simulink model "Cathode_Simscape_Model"  (R2023a)
settings: Solver=VariableStepAuto  StartTime=0.0  StopTime=500  RelTol=1e-3
undefined symbols (not defined in the file or in its folder): sigbuilder_block
libraries: fl_lib x55, nesl_utility x45, SimscapeFluids_lib x15
(part 1 of 3)
settings Model: Creator=mahesh.kumar  LastModifiedBy=mahesh.kumar

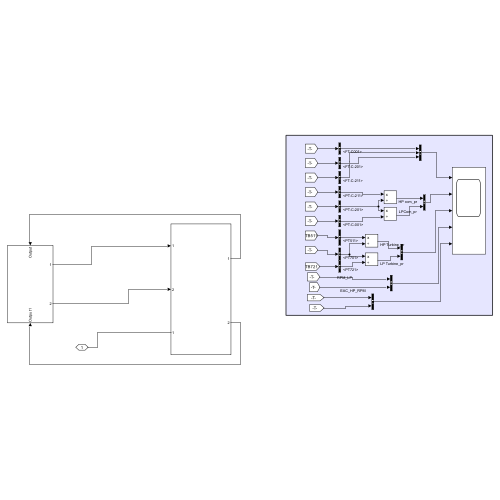
[thumbnail: Simulink's stored preview of the top-level diagram]
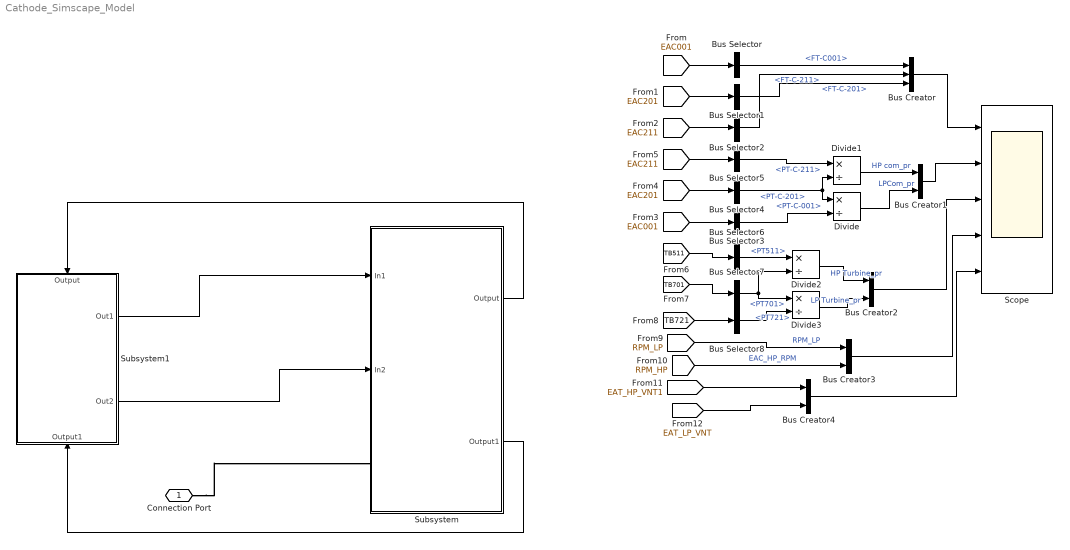
== system Cathode_Simscape_Model ==
  Bus Creator : BusCreator  Inputs=3
  Bus Creator{1..4} (4 alike) : BusCreator  Inputs=2
  Bus Selector : BusSelector  OutputSignals=FT-C001
  Bus Selector1 : BusSelector  OutputSignals=FT-C-201
  Bus Selector2 : BusSelector  OutputSignals=FT-C-211
  Bus Selector3 : BusSelector  OutputSignals=PT-C-001
  Bus Selector4 : BusSelector  OutputSignals=PT-C-201
  Bus Selector5 : BusSelector  OutputSignals=PT-C-211
  Bus Selector6 : BusSelector  OutputSignals=PT511
  Bus Selector7 : BusSelector  OutputSignals=PT701
  Bus Selector8 : BusSelector  OutputSignals=PT721
  Divide{,1..3} (4 alike) : Product  Inputs=*/
  Scope : Scope  NumInputPorts=5
  Subsystem : Subsystem
  Subsystem1 : Subsystem
      settings: PortSchema="{\"entries\":[{\"content\":{\"sides\":[{\"content\":{},\"type\":\"ConnectorPlacement.EquallySpacedRectSide\",\"uuid\":\"984249b6-2700-4899-8357-f545c62d10ef\"},{\"content\":{\"connectorIds\":[\"Out1\",\"Out2\"],\"side\":\"RIGHT\"},\"type\":\"ConnectorPlacement.EquallySpacedRectSide\",\"uuid\":\"0a8907d5-2e85-49aa-bb23-8dd611067149\"},{\"content\":{\"connectorIds\":[\"In1\"],\"side\":\"TOP\"},\"type\":\"ConnectorPlacement.EquallySpacedRectSide\",\"uuid\":\"e00e54d0-6dbf-429f-9506-ec6eaddd1938\"},{\"content\":{\"connectorIds\":[\"In2\"],\"side\":\"BOTTOM\"},\"type\":\"ConnectorPlacement.EquallySpacedRectSide\",\"uuid\":\"b22db3dd-63f8-4b6d-a56a-cf8370c91cba\"}]},\"type\":\"ConnectorPlacement.EquallySpacedConnector\",\"uuid\":\"9582d771-9072-4842-b99f-8327be8cf876\"}],\"packageUris\":[\"http://schema.mathworks.com/mf0/Connector/R2020b\"],\"version\":\"1.0\"}"
  Connection Port : PMIOPort  Side=Left
  wires:
  Subsystem1/1(Out1) -> Subsystem/1(In1)
  Subsystem1/2(Out2) -> Subsystem/2(In2)
  Subsystem/1(Output) -> Subsystem1/1(Output)
  [EAC001] -> Bus Selector/1
  [EAC201] -> Bus Selector1/1
  [EAC211] -> Bus Selector2/1
  Bus Selector/1 -> Bus Creator/1  "<FT-C001>"
  Bus Selector1/1 -> Bus Creator/3  "<FT-C-201>"
  Bus Selector2/1 -> Bus Creator/2  "<FT-C-211>"
  Bus Selector4/1 -> Divide/1, Divide1/2  "<PT-C-201>"
  [EAC001] -> Bus Selector3/1
  [EAC201] -> Bus Selector4/1
  Bus Selector3/1 -> Divide/2  "<PT-C-001>"
  [EAC211] -> Bus Selector5/1
  Bus Selector5/1 -> Divide1/1  "<PT-C-211>"
  Divide1/1 -> Bus Creator1/1  "HP com_pr"
  Divide/1 -> Bus Creator1/2  "LPCom_pr"
  [TB511] -> Bus Selector6/1
  [TB701] -> Bus Selector7/1
  Bus Selector6/1 -> Divide2/1  "<PT511>"
  Bus Selector7/1 -> Divide3/1, Divide2/2  "<PT701>"
  [TB721] -> Bus Selector8/1
  Bus Selector8/1 -> Divide3/2  "<PT721>"
  Divide2/1 -> Bus Creator2/1  "HP Turbine_pr"
  Divide3/1 -> Bus Creator2/2  "LP Turbine_pr"
  Subsystem/2(Output1) -> Subsystem1/2(Output1)
  Bus Creator/1 -> Scope/1
  Bus Creator1/1 -> Scope/2
  Bus Creator2/1 -> Scope/3
  [RPM_LP] -> Bus Creator3/1  "RPM_LP"
  [RPM_HP] -> Bus Creator3/2  "EAC_HP_RPM"
  Bus Creator3/1 -> Scope/4
  [EAT_HP_VNT1] -> Bus Creator4/1
  [EAT_LP_VNT] -> Bus Creator4/2
  Bus Creator4/1 -> Scope/5
  connections:
  Connection Port/RConn1 -- Subsystem/LConn1

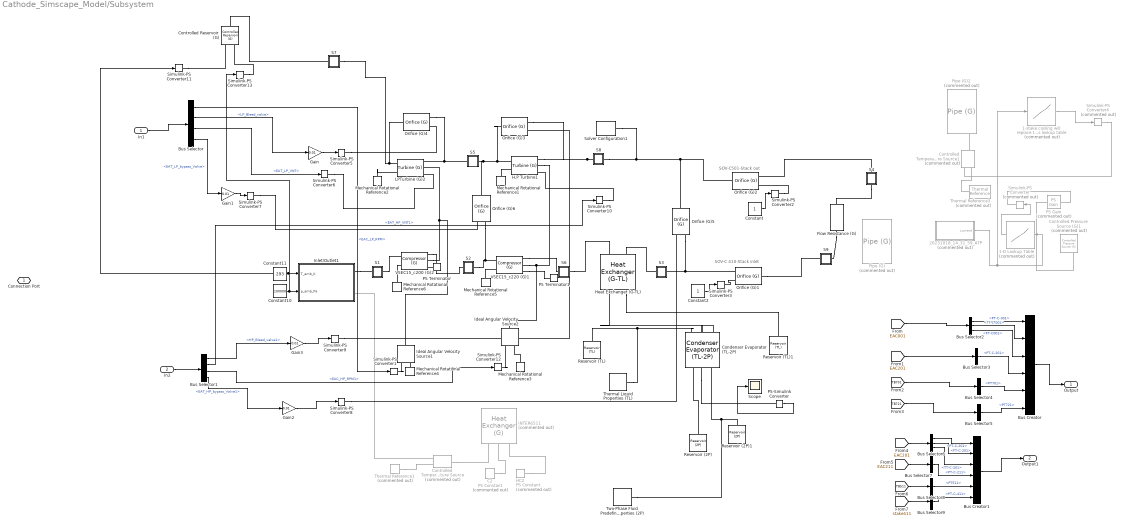
== system Cathode_Simscape_Model/Subsystem ==
  note: SOV-C 410-Stack inlet
  note: SOV-C501-Stack out
  In1 : Inport
  In2 : Inport  Port=2
  1-D Lookup Table : Lookup_n-D  Commented=on  NumberOfTableDimensions=1  BreakpointsForDimension1=[50;100;150;200;250;300;350;400;450;500;550;600]  Table=[49.4;55;69.9;83;109;105;153;173;174;220;230;0]  InternalRulePriority=Speed  RndMeth=Simplest
  1-stake cooling will replace this lookup table : Lookup_n-D  Commented=on  NumberOfTableDimensions=1  BreakpointsForDimension1=[0;50;100;200;400]  Table=[312;322;332;342;352]  InternalRulePriority=Speed  RndMeth=Simplest
  20231018_14_31_59_ATP : Subsystem  Tag=STV Subsys  Commented=on  LoadFcn=sigbuilder_block('load');  StartFcn=sigbuilder_block('start');  StopFcn=sigbuilder_block('stop');  ClipboardFcn=sigbuilder_block('clipboard');  mask(Sigbuilder block){tuvar=[0:10]}
      mask help: Simulink:masks:SigbuilderBlock_MD
      mask init:
      | if ~strcmp(get_param(bdroot(gcbh),'SimulationStatus'),'stopped') tuvar = sigbuilder_block('maskInit'); end
      settings: CopyFcn=sigbuilder_block('copy');  DeleteFcn=sigbuilder_block('delete');  ModelCloseFcn=sigbuilder_block('modelClose');  PreSaveFcn=sigbuilder_block('preSave');  PauseFcn=sigbuilder_block('pause');  ContinueFcn=sigbuilder_block('continue');  NameChangeFcn=sigbuilder_block('namechange');  OpenFcn=sigbuilder_block('open',[368.25 148.5 938.25 516 ]);  CloseFcn=sigbuilder_block('close');
      mask Display: plot(0, 0, 100, 100,[2, 2, 32, 32, 2], [68, 8, 8, 68, 68],[32, 2], [38, 38], [32, 19, 2],[53, 60, 44], [32, 17, 17, 2],[16, 16, 31, 31]);txt = getActiveGroup(gcbh);text(2, 100, txt,'verticalAlignment', 'top');
  Bus Creator : BusCreator  Inputs=6
  Bus Creator1 : BusCreator  Inputs=6
  Bus Selector : BusSelector  OutputSignals=EAC_LP_RPM,LP_Bleed_valve,EAT_LP_VNT,EAT_LP_bypass_Valve
  Bus Selector1 : BusSelector  OutputSignals=HP_Bleed_valve1,EAT_HP_VNT1,EAC_HP_RPM1,EAT_HP_bypass_Valve1
  Bus Selector2 : BusSelector  OutputSignals=PT-C-001,TT-C-001,FT-C001
  Bus Selector3 : BusSelector  OutputSignals=PT-C-201
  Bus Selector4 : BusSelector  OutputSignals=PT701
  Bus Selector5 : BusSelector  OutputSignals=PT721
  Bus Selector6 : BusSelector  OutputSignals=PT-C-201,FT-C-201,TT-C-201
  Bus Selector7 : BusSelector  OutputSignals=PT-C-211
  Bus Selector8 : BusSelector  OutputSignals=PT511
  Bus Selector9 : BusSelector  OutputSignals=PT-C-411
  C2 : fl_lib/Physical Signals/Sources/PS Constant  Commented=on  constant=12361
  Condenser Evaporator (TL-2P) : SimscapeFluids_lib/Fluid Network Interfaces/Heat Exchangers/Condenser Evaporator (TL-2P)  flow_arrangement=fluids.interfaces.heat_exchangers.enum.FlowArrangementTL2P.Cross  cross_flow_arrangement=fluids.interfaces.heat_exchangers.enum.CrossFlowArrangementTL2P.UnmixedUnmixed  R_wall=0 K/kW  area_A1=0.01 m^2  area_B1=0.01 m^2  area_A2=0.01 m^2  area_B2=0.01 m^2  flow_geometry_TL=fluids.interfaces.heat_exchangers.enum.FlowGeometryTL.InsideTubes  tube_num_TL=25  tube_length_TL=1 m  tube_cross_section_TL=fluids.interfaces.heat_exchangers.enum.TubeCrossSection.Circular  tube_diameter_TL=0.05 m  tube_width_TL=0.05 m  tube_height_TL=0.05 m  tube_inner_diameter_TL=0.05 m  tube_outer_diameter_TL=0.1 m  tube_flow_area_TL=0.002 m^2  tube_wetted_perimeter_TL=0.15 m  tube_heat_perimeter_TL=0.15 m  tube_pressure_loss_spec_TL=fluids.interfaces.heat_exchangers.enum.TubePressureLossSpec.Haaland  tube_loss_coeff_TL=10  tube_local_pressure_loss_spec_TL=fluids.thermal_liquid.pipes_fittings.enum.LocalLossSpec.AggregateLength  tube_length_add_TL=0.1 m  tube_local_loss_coefficient_TL=0.1  tube_roughness_pressure_TL=15e-6 m  tube_Re_lam_pressure_TL=2000  tube_Re_tur_pressure_TL=4000  tube_shape_factor_generic_TL=64  tube_heat_coeff_spec_TL=fluids.interfaces.heat_exchangers.enum.TubeHeatCoeffSpec.Gneilinski  tube_colburn_coeff_TL=[.023, .8, .33]  tube_roughness_heat_TL=15e-6 m  tube_Re_lam_heat_TL=2000  tube_Re_tur_heat_TL=4000  tube_Nu_lam_generic_TL=3.66  bank_arrangement_TL=fluids.interfaces.heat_exchangers.enum.BankArrangement.Inline  bank_num_rows_TL=5  bank_tubes_per_row_TL=5  bank_width_TL=1 m  bank_tube_diameter_TL=0.05 m  bank_longitudinal_pitch_TL=0.15 m  bank_transverse_pitch_TL=0.15 m  bank_pressure_loss_spec_TL=fluids.interfaces.heat_exchangers.enum.BankPressureLossSpec.Martin  bank_euler_TL=10  bank_heat_coeff_spec_TL=fluids.interfaces.heat_exchangers.enum.BankHeatCoeffSpec.Martin  bank_colburn_coeff_TL=[.27, .63, .36]  generic_flow_area_TL=0.01 m^2  generic_heat_area_TL=2 m^2  generic_volume_TL=0.05 m^3  generic_loss_coeff_TL=10  generic_colburn_coeff_TL=[.023, .8, .33]  fouling_factor_TL=0.1 K*m^2/kW  fin_area_TL=0 m^2  fin_efficiency_TL=0.5  p_init_TL=0.101325 MPa  T_init_TL=293.15 K  tube_num_2P=25  tube_length_2P=1 m  tube_cross_section_2P=fluids.interfaces.heat_exchangers.enum.TubeCrossSection.Circular  tube_diameter_2P=0.05 m  tube_width_2P=0.05 m  tube_height_2P=0.05 m  tube_inner_diameter_2P=0.05 m  tube_outer_diameter_2P=0.1 m  tube_flow_area_2P=0.002 m^2  tube_wetted_perimeter_2P=0.15 m  tube_heat_perimeter_2P=0.15 m  tube_pressure_loss_spec_2P=fluids.interfaces.heat_exchangers.enum.TubePressureLossSpec2P.Haaland  tube_loss_coeff_2P=10  tube_local_pressure_loss_spec_2P=fluids.two_phase_fluid.pipes_fittings.enum.LocalLossSpec.AggregateLength  tube_length_add_2P=0.1 m  tube_local_loss_coefficient_2P=0.1  tube_roughness_pressure_2P=15e-6 m  tube_Re_lam_pressure_2P=2000  tube_Re_tur_pressure_2P=4000  tube_shape_factor_generic_2P=64  tube_heat_coeff_spec_2P=fluids.interfaces.heat_exchangers.enum.TubeHeatCoeffSpec2P.GneilinskiCavalliniZecchin  tube_colburn_coeff_liq_2P=[.023, .8, .33]  tube_colburn_coeff_mix_2P=[.05, .8, .33]  tube_colburn_coeff_vap_2P=[.023, .8, .33]  tube_roughness_heat_2P=15e-6 m  tube_Re_lam_heat_2P=2000  tube_Re_tur_heat_2P=4000  tube_Nu_lam_generic_2P=3.66  fouling_factor_2P=0.1 K*m^2/kW  fin_area_2P=0 m^2  fin_efficiency_2P=0.5  energy_spec_2P=foundation.enum.energy_spec.temperature  p_init_2P=0.101325 MPa  T_init_2P=293.15 K  x_init_2P=0.5  alpha_init_2P=0.5  h_init_2P=1500 kJ/kg  u_init_2P=1500 kJ/kg
      settings: InternalSimscapePortConfiguration="{\"Bottom\":[],\"Left\":[{\"id\":\"A1\",\"label\":\"A1\",\"type\":\"foundation.thermal_liquid.thermal_liquid\"},{\"id\":\"B1\",\"label\":\"B1\",\"type\":\"foundation.thermal_liquid.thermal_liquid\"}],\"Right\":[{\"id\":\"A2\",\"label\":\"A2\",\"type\":\"foundation.two_phase_fluid.two_phase_fluid\"},{\"id\":\"B2\",\"label\":\"B2\",\"type\":\"foundation.two_phase_fluid.two_phase_fluid\"}],\"Top\":[{\"id\":\"Z\",\"label\":\"Z\",\"type\":\"output\"}]}"
  Constant : Constant
  Constant10 : Constant  Value=100000
  Constant11 : Constant  Value=293
  Constant2 : Constant
  Controlled Temperature Source : fl_lib/Thermal/Thermal Sources/Controlled Temperature Source  Commented=on
  Controlled Temperature Source1 : fl_lib/Thermal/Thermal Sources/Controlled Temperature Source  Commented=on
  Controlled Pressure Source (G)1 : fl_lib/Gas/Sources/Controlled Pressure Source (G)  Commented=on  power_spec=foundation.enum.power_spec.none  area_A=0.01 m^2  area_B=0.01 m^2
      settings: InternalSimscapePortConfiguration="{\"Bottom\":[],\"Left\":[{\"id\":\"A\",\"label\":\"A\",\"type\":\"foundation.gas.gas\"},{\"id\":\"P\",\"label\":\"P\",\"type\":\"input\"}],\"Right\":[{\"id\":\"B\",\"label\":\"B\",\"type\":\"foundation.gas.gas\"}],\"Top\":[]}"
  Controlled Reservoir (G) : fl_lib/Gas/Elements/Controlled Reservoir (G)  area_A=0.002 m^2
      settings: InternalSimscapePortConfiguration="{\"Bottom\":[],\"Left\":[{\"id\":\"A\",\"label\":\"A\",\"type\":\"foundation.gas.gas\"}],\"Right\":[{\"id\":\"T_in\",\"label\":\"T\",\"type\":\"input\"},{\"id\":\"p_in\",\"label\":\"P\",\"type\":\"input\"}],\"Top\":[]}"
  Flow Resistance (G) : fl_lib/Gas/Elements/Flow Resistance (G)  delta_p_nominal=20000 Pa  mdot_nominal=0.1 kg/s  rho_nominal=0 kg/m^3  area=0.002 m^2  laminar_fraction=1e-3
      settings: InternalSimscapePortConfiguration="{\"Bottom\":[],\"Left\":[{\"id\":\"A\",\"label\":\"A\",\"type\":\"foundation.gas.gas\"}],\"Right\":[{\"id\":\"B\",\"label\":\"B\",\"type\":\"foundation.gas.gas\"}],\"Top\":[]}"
  Gain{,1..3} (4 alike) : Gain  Gain=0.01
  H.P Turbine1 : SimscapeFluids_lib/Gas/Turbomachinery/Turbine (G)  parameterization=fluids.gas.turbomachinery.enum.TurbineParameterization.Tabulated1D  omega_TLU_2="[40000, 60000, 80000,  100000, 120000] rpm"  variable_nozzle=true  min_nozzle_opening=1e-3  max_nozzle_opening=1  pr_nom=2  mdot_nom=48 kg/s  pr_mdot_TLU=[1.02750530846485, 1.10195466284075, 1.21807977044476, 1.39993572453372, 1.59797761836442, 1.85853658536585]  mdot_TLU=[37.7618364418938, 59.6556671449067, 79.3400286944046, 95.2080344332855, 105.652797704448, 112.682926829268] g/s  pr_mdot_TLU_2=|  mdot_TLU_2=|  efficiency_constant=0.8  pr_eta_TLU=[1.02750530846485, 1.10195466284075, 1.21807977044476, 1.39993572453372, 1.59797761836442, 1.85853658536585]  eta_TLU=[0.500,0.473,0.375,0.337,0.310,0.290]  pr_eta_TLU_2=|  eta_TLU_2=|  p_reference=1 bar  T_reference=293 K  mechanical_efficiency=0.98  area_A=0.002 m^2  area_B=0.002 m^2
      pr_mdot_TLU_2=|
      | [1.02750530846485 1.10195466284075 1.21807977044476 1.39993572453372 1.59797761836442 1.85853658536585;
      | 1.04528436154950 1.18521664275466 1.44373486370158 1.67865939741750 1.86888723098996 2.13912883787661; 
      | 1.05182209469154 1.19671965566714 1.42019626972740 1.67269325681492 1.95725911047346 2.27246599713056; 
      | 1.05523558106169 1.20345710186514 1.43823012912482 1.69874777618364 1.91463070301291 2.21694806312769; 
      | 1.06813888091822 1.31716040172166 1.53931248206600 1.75356786226686 2.00627144906743 2.20147144906743]
      mdot_TLU_2=|
      | [37.7618364418938 59.6556671449067 79.3400286944046 95.2080344332855 105.652797704448 112.682926829268;
      | 32.5394548063128 57.8479196556671 77.7331420373027 85.7675753228121 90.7890961262554 95.4088952654233; 
      | 28.5222381635581 49.0100430416069 64.2754662840746 73.1133428981349 79.9426111908178 79.7417503586801; 
      | 22.2955523672884 39.1678622668580 51.6212338593974 59.8565279770445 63.2711621233860 65.6814921090387; 
      | 19.2826398852224 36.1549497847920 43.3859397417504 47.6040172166428 50.4160688665710 50.4160688665710] g/s
      pr_eta_TLU_2=|
      | [1.02750530846485 1.10195466284075 1.21807977044476 1.39993572453372 1.59797761836442 1.85853658536585;
      | 1.04528436154950 1.18521664275466 1.44373486370158 1.67865939741750 1.86888723098996 2.13912883787661; 
      | 1.05182209469154 1.19671965566714 1.42019626972740 1.67269325681492 1.95725911047346 2.27246599713056; 
      | 1.05523558106169 1.20345710186514 1.43823012912482 1.69874777618364 1.91463070301291 2.21694806312769; 
      | 1.06813888091822 1.31716040172166 1.53931248206600 1.75356786226686 2.00627144906743 2.20147144906743]
      eta_TLU_2=|
      | [0.7 0.7 0.7 0.7 0.7 0.7;
      |   0.7 0.7 0.7 0.7 0.7 0.7;
      |    0.7 0.7 0.7 0.7 0.7 0.7;
      |    0.7 0.7 0.7 0.7 0.7 0.7 ;  0.7 0.7 0.7 0.7 0.7 0.7 ]
      settings: InternalSimscapePortConfiguration="{\"Bottom\":[],\"Left\":[{\"id\":\"A\",\"label\":\"A\",\"type\":\"foundation.gas.gas\"},{\"id\":\"R\",\"label\":\"R\",\"type\":\"foundation.mechanical.rotational.rotational\"},{\"id\":\"VN\",\"label\":\"VN\",\"type\":\"input\"}],\"Right\":[{\"id\":\"B\",\"label\":\"B\",\"type\":\"foundation.gas.gas\"},{\"id\":\"C\",\"label\":\"C\",\"type\":\"foundation.mechanical.rotational.rotational\"}],\"Top\":[]}"
  HC2 : fl_lib/Physical Signals/Sources/PS Constant  Commented=on  constant=3981.072
  Heat Exchanger (G-TL) : SimscapeFluids_lib/Fluid Network Interfaces/Heat Exchangers/Heat Exchanger (G-TL)  hex_type=fluids.interfaces.enum.flow_arrangement_spec.parallel_counter  shell_num=1  cross_type=fluids.interfaces.enum.cross_flow_heat_exchanger_G_TL_spec.mixed_mixed  NTU_TLU=[.5, 1, 2, 3, 4, 5]  CR_TLU=[0, .25, .5, .75, 1]  eff_TLU=[.3, .3, .3, .3, .3; .6, .55, .5, .47, .43; .85, .76, .68, .61, .55; .94, .83, .72, .65, .58; .98, .86, .75, .66, .58; .99, .86, .75, .66, .58]  wall_thermal_dynamics=simscape.enum.onoff.off  thermal_mass_wall=447 J/K  R_wall=1.6e-4 K/W  min_flow_area_1=0.01 m^2  Dh_press_1=0.1 m  gas_volume_1=0.01 m^3  Re_lam_1=2000  Re_tur_1=4000  pressure_loss_spec_1=fluids.interfaces.enum.pressure_loss_spec.constant  pressure_loss_coeff_1=0.1  length_press_1=1 m  length_add_1=0.1 m  roughness_1=15e-6 m  Re_friction_TLU_1=[400, 1000, 1500, 3000, 4000, 6000, 10000, 20000, 40000, 60000, 100000, 100000000]  friction_factor_TLU_1=[.264, .112, .071, .0417, .0387, .0268, .025, .0232, .0226, .022, .0214, .0214]  shape_factor_1=64  Re_Euler_TLU_1=[50, 500, 1000, 2000]  Euler_TLU_1=[4.4505, .6864, .4791, .3755]  heat_transfer_spec_1=fluids.interfaces.enum.heat_transfer_spec.constant  heat_transfer_area_1=0.4 m^2  heat_coeff_1=100 W/(K*m^2)  length_heat_1=1 m  Nu_lam_1=3.66  Re_Colburn_TLU_1=[100, 150, 1000]  Colburn_factor_TLU_1=[.019, .013, .002]  Re_Nu_TLU_1=[100, 150, 1000]  Pr_Nu_TLU_1=[1, 10]  Nu_TLU_1=[3.72, 4.21; 3.75, 4.44; 4.21, 7.15]  fouling_factor_1=1e-4 K*m^2/W  mdot_threshold_1=1e-6 kg/s  min_heat_coeff_1=5 W/(K*m^2)  min_flow_area_2=0.00075 m^2  Dh_press_2=0.1 m  liquid_volume_2=0.01 m^3  Re_lam_2=2000  Re_tur_2=4000  pressure_loss_spec_2=fluids.interfaces.enum.pressure_loss_spec.constant  pressure_loss_coeff_2=0.1  length_press_2=1 m  length_add_2=0.1 m  roughness_2=15e-6 m  Re_friction_TLU_2=[400, 1000, 1500, 3000, 4000, 6000, 10000, 20000, 40000, 60000, 100000, 100000000]  friction_factor_TLU_2=[.264, .112, .071, .0417, .0387, .0268, .025, .0232, .0226, .022, .0214, .0214]  shape_factor_2=64  Re_Euler_TLU_2=[50, 500, 1000, 2000]  Euler_TLU_2=[4.4505, .6864, .4791, .3755]  heat_transfer_spec_2=fluids.interfaces.enum.heat_transfer_spec.constant  heat_transfer_area_2=0.4 m^2  heat_coeff_2=100 W/(K*m^2)  length_heat_2=1 m  Nu_lam_2=3.66  Re_Colburn_TLU_2=[100, 150, 1000]  Colburn_factor_TLU_2=[.019, .013, .002]  Re_Nu_TLU_2=[100, 150, 1000]  Pr_Nu_TLU_2=[1, 10]  Nu_TLU_2=[3.72, 4.21; 3.75, 4.44; 4.21, 7.15]  fouling_factor_2=1e-4 K*m^2/W  min_heat_coeff_2=5 W/(K*m^2)  T0_1=293.15 K  p0_1=0.101325 MPa  dynamic_compressibility_2=simscape.enum.onoff.on  T0_2=293.15 K  p0_2=0.101325 MPa  mdot1_TLU=[.3, .5, .6, .7, 1, 1.4, 1.9, 2.3] kg/s  mdot2_TLU=[.3, .5, 1, 1.3, 1.7, 2, 2.6, 3.3] kg/s  SD_TLU=[.324, .3533, .404, .4253, .4333, .4373, .4453, .4533; .3813, .424, .496, .5307, .544, .5547, .5693, .5787; .4267, .4827, .5813, .6173, .6413, .6573, .672, .6827; .4613, .528, .64, .6987, .7267, .7467, .7707, .7853; .5533, .6467, .8227, .928, .9853, 1.0187, 1.0653, 1.0973; .58, .688, .8853, 1.0147, 1.08, 1.124, 1.176, 1.2147; .624, .7467, .992, 1.148, 1.244, 1.304, 1.3773, 1.4267; .656, .7907, 1.0667, 1.26, 1.376, 1.452, 1.548, 1.612] kW/K  Q_check=fluids.interfaces.enum.SD_max_check.warning  mdot_dp_TLU_1=[.3, .5, 1, 1.5, 2, 2.5] kg/s  p_diff_TLU_1=[3, 5, 10, 25, 35, 50] * 1e-3 MPa  T_ref_in_1=293.15 K  p_ref_in_1=0.101325 MPa  area_1=0.01 m^2  mdot_dp_TLU_2=[.3, .5, 1, 1.5, 2, 2.5] kg/s  p_diff_TLU_2=[3, 5, 10, 25, 35, 50] * 1e-3 MPa  T_ref_in_2=293.15 K  p_ref_in_2=0.101325 MPa  mdot_threshold_2=1e-3 kg/s  area_2=0.01 m^2
      settings: InternalSimscapePortConfiguration="{\"Bottom\":[],\"Left\":[{\"id\":\"A1\",\"label\":\"A1\",\"type\":\"foundation.gas.gas\"},{\"id\":\"B1\",\"label\":\"B1\",\"type\":\"foundation.gas.gas\"}],\"Right\":[{\"id\":\"A2\",\"label\":\"A2\",\"type\":\"foundation.thermal_liquid.thermal_liquid\"},{\"id\":\"B2\",\"label\":\"B2\",\"type\":\"foundation.thermal_liquid.thermal_liquid\"}],\"Top\":[]}"
  INTER6511 : SimscapeFluids_lib/Fluid Network Interfaces/Heat Exchangers/Heat Exchanger (G)  Commented=on  hex_type=fluids.interfaces.enum.flow_arrangement_spec.cross_flow  shell_num=1  cross_type=fluids.interfaces.enum.cross_flow_heat_exchanger_G_spec.unmixed_mixed  NTU_TLU=[.5, 1, 2, 3, 4, 5]  CR_TLU=[0, .25, .5, .75, 1]  eff_TLU=[.3, .3, .3, .3, .3; .6, .55, .5, .47, .43; .85, .76, .68, .61, .55; .94, .83, .72, .65, .58; .98, .86, .75, .66, .58; .99, .86, .75, .66, .58]  R_wall=0.00016331 K/W  min_flow_area_1=.00075 m^2  Dh_press_1=0.0028302 m  gas_volume_1=0.0003375 m^3  Re_lam_1=2000  Re_tur_1=4000  pressure_loss_spec_1=fluids.interfaces.enum.pressure_loss_spec.constant  pressure_loss_coeff_1=0.05  length_press_1=1 m  length_add_1=0.1 m  roughness_1=15e-6 m  Re_friction_TLU_1=[400, 1000, 1500, 3000, 4000, 6000, 10000, 20000, 40000, 60000, 100000, 100000000]  friction_factor_TLU_1=[.264, .112, .071, .0417, .0387, .0268, .025, .0232, .0226, .022, .0214, .0214]  shape_factor_1=64  Re_Euler_TLU_1=[50, 500, 1000, 2000]  Euler_TLU_1=[4.4505, .6864, .4791, .3755]  heat_transfer_spec_1=fluids.interfaces.enum.heat_transfer_spec.constant  heat_transfer_area_1=0.45 m^2  heat_coeff_1=405 W/(K*m^2)  length_heat_1=1 m  Nu_lam_1=3.66  Re_Colburn_TLU_1=[100, 150, 1000]  Colburn_factor_TLU_1=[.019, .013, .002]  Re_Nu_TLU_1=[100, 150, 1000]  Pr_Nu_TLU_1=[1, 10]  Nu_TLU_1=[3.72, 4.21; 3.75, 4.44; 4.21, 7.15]  fouling_factor_1=1e-4 K*m^2/W  mdot_threshold_1=1e-6 kg/s  min_heat_coeff_1=5 W/(K*m^2)  heat_transfer_area_2=3 m^2  fouling_factor_2=0 K*m^2/W  min_heat_coeff_2=0.01 W/(K*m^2)  T0_1=20 degC  p0_1=0.1 MPa  mdot1_TLU=[.3, .5, .6, .7, 1, 1.4, 1.9, 2.3] kg/s  mdot2_TLU=[.3, .5, 1, 1.3, 1.7, 2, 2.6, 3.3] kg/s  SD_TLU=[.324, .3533, .404, .4253, .4333, .4373, .4453, .4533; .3813, .424, .496, .5307, .544, .5547, .5693, .5787; .4267, .4827, .5813, .6173, .6413, .6573, .672, .6827; .4613, .528, .64, .6987, .7267, .7467, .7707, .7853; .5533, .6467, .8227, .928, .9853, 1.0187, 1.0653, 1.0973; .58, .688, .8853, 1.0147, 1.08, 1.124, 1.176, 1.2147; .624, .7467, .992, 1.148, 1.244, 1.304, 1.3773, 1.4267; .656, .7907, 1.0667, 1.26, 1.376, 1.452, 1.548, 1.612] kW/K  Q_check=fluids.interfaces.enum.SD_max_check.warning  mdot_dp_TLU_1=[.3, .5, 1, 1.5, 2, 2.5] kg/s  p_diff_TLU_1=[3, 5, 10, 25, 35, 50] * 1e-3 MPa  T_ref_in_1=293.15 K  p_ref_in_1=0.101325 MPa  area_1=0.01 m^2
      settings: InternalSimscapePortConfiguration="{\"Bottom\":[],\"Left\":[{\"id\":\"A1\",\"label\":\"A1\",\"type\":\"foundation.gas.gas\"},{\"id\":\"B1\",\"label\":\"B1\",\"type\":\"foundation.gas.gas\"}],\"Right\":[{\"id\":\"H2\",\"label\":\"H2\",\"type\":\"foundation.thermal.thermal\"},{\"id\":\"C2\",\"label\":\"C2\",\"type\":\"input\"},{\"id\":\"HC2\",\"label\":\"HC2\",\"type\":\"input\"}],\"Top\":[]}"
  Ideal Angular Velocity Source1 : fl_lib/Mechanical/Mechanical Sources/Ideal Angular Velocity Source
  Ideal Angular Velocity Source2 : fl_lib/Mechanical/Mechanical Sources/Ideal Angular Velocity Source
  Inlet/Outlet1 : Subsystem
  LPTurbine (G)2 : SimscapeFluids_lib/Gas/Turbomachinery/Turbine (G)  parameterization=fluids.gas.turbomachinery.enum.TurbineParameterization.Tabulated1D  omega_TLU_2=[5000, 6000, 7000, 8000, 9000, 10000, 11000] rpm  variable_nozzle=true  min_nozzle_opening=1e-3  max_nozzle_opening=1  pr_nom=2  mdot_nom=48 kg/s  pr_mdot_TLU="[1.03,\t1.07,\t1.12,\t1.18,\t1.26,\t1.38,\t1.52,\t1.66,\t1.76]"  mdot_TLU="[44.61,\t65.49,\t83.78,\t102.00,\t118.06,\t131.34,\t141.85,\t149.18,\t151.56] g/s"  pr_mdot_TLU_2=[1.217, 1.285, 1.323, 1.363, 1.402, 1.427, 1.495, 1.545, 1.6, 1.687, 1.747, 1.8074; 1.231, 1.302, 1.356, 1.404, 1.443, 1.473, 1.525, 1.577, 1.635, 1.709, 1.782, 1.845; 1.242, 1.328, 1.388, 1.437, 1.528, 1.617, 1.704, 1.811, 1.915, 1.979, 2.053, 2.1226; 1.244, 1.339, 1.417, 1.465, 1.528, 1.584, 1.692, 1.787, 1.899, 2, 2.075, 2.1492; 1.245, 1.34, 1.425, 1.492, 1.546, 1.684, 1.748, 1.882, 1.987, 2.084, 2.167, 2.2458; 1.251, 1.345, 1.442, 1.521, 1.596, 1.692, 1.849, 1.972, 2.1, 2.173, 2.259, 2.3424; 1.248, 1.348, 1.447, 1.516, 1.581, 1.651, 1.749, 1.839, 1.93, 2.024, 2.154, 2.242]  mdot_TLU_2=[40.403, 44.417, 46.653, 47.966, 48.97, 49.544, 50.001, 50.081, 50.086, 50.095, 50.09, 50.0922; 40.044, 43.754, 46.125, 47.626, 48.513, 49.105, 49.481, 49.58, 49.597, 49.624, 49.638, 49.633; 39.941, 43.795, 46.017, 47.335, 48.795, 49.199, 49.279, 49.27, 49.248, 49.23, 49.255, 49.2428; 39.896, 43.512, 45.914, 47.061, 48.011, 48.558, 48.943, 49.042, 49.069, 49.01, 49.046, 49.0266; 39.524, 42.934, 45.686, 46.743, 47.715, 48.67, 48.777, 48.836, 48.876, 48.836, 48.845, 48.8184; 39.439, 43.01, 45.556, 46.801, 47.792, 48.388, 48.634, 48.67, 48.639, 48.647, 48.625, 48.5912; 39.502, 42.849, 45.336, 46.385, 47.312, 47.877, 48.222, 48.397, 48.459, 48.482, 48.455, 48.414] kg/s  efficiency_constant=0.8  pr_eta_TLU="[1.03,\t1.07,\t1.12,\t1.18,\t1.26,\t1.38,\t1.52,\t1.66,\t1.76]"  eta_TLU="[0.050, \t0.325, \t0.520, \t0.550, \t0.610, \t0.600, \t0.590, \t0.580, \t0.575]"  pr_eta_TLU_2=[1.224, 1.246, 1.292, 1.387, 1.457, 1.534, 1.61, 1.686, 1.743, 1.79, 1.871, 1.914; 1.237, 1.25, 1.28, 1.369, 1.459, 1.553, 1.629, 1.716, 1.799, 1.846, 1.927, 1.97; 1.241, 1.255, 1.283, 1.326, 1.401, 1.509, 1.591, 1.704, 1.806, 1.913, 1.994, 2.037; 1.25, 1.265, 1.308, 1.364, 1.456, 1.532, 1.637, 1.739, 1.851, 1.934, 2.042, 2.085; 1.281, 1.314, 1.371, 1.425, 1.498, 1.574, 1.647, 1.749, 1.878, 1.979, 2.091, 2.18; 1.252, 1.328, 1.425, 1.544, 1.642, 1.757, 1.873, 2.005, 2.1, 2.204, 2.248, 2.28; 1.382, 1.43, 1.495, 1.586, 1.688, 1.791, 1.887, 1.99, 2.079, 2.158, 2.249, 2.36]  eta_TLU_2=[.72, .754, .759, .739, .714, .679, .643, .603, .554, .524, .494, .48; .716, .757, .794, .819, .812, .788, .761, .728, .692, .662, .632, .618; .629, .691, .775, .831, .858, .869, .859, .842, .816, .782, .752, .738; .594, .668, .757, .804, .857, .883, .892, .893, .884, .865, .835, .821; .664, .72, .779, .823, .858, .883, .897, .905, .904, .896, .883, .868; .559, .61, .673, .741, .788, .835, .869, .895, .908, .899, .854, .751; .718, .785, .824, .855, .882, .9, .908, .906, .884, .857, .804, .701]  p_reference=1 bar  T_reference=293 K  mechanical_efficiency=0.98  area_A=0.002 m^2  area_B=0.002 m^2
      settings: InternalSimscapePortConfiguration="{\"Bottom\":[],\"Left\":[{\"id\":\"A\",\"label\":\"A\",\"type\":\"foundation.gas.gas\"},{\"id\":\"R\",\"label\":\"R\",\"type\":\"foundation.mechanical.rotational.rotational\"},{\"id\":\"VN\",\"label\":\"VN\",\"type\":\"input\"}],\"Right\":[{\"id\":\"B\",\"label\":\"B\",\"type\":\"foundation.gas.gas\"},{\"id\":\"C\",\"label\":\"C\",\"type\":\"foundation.mechanical.rotational.rotational\"}],\"Top\":[]}"
  Mechanical Rotational Reference{1..6} (6 alike) : fl_lib/Mechanical/Rotational Elements/Mechanical Rotational Reference
  Orifice (G){1..6} (6 alike) : SimscapeFluids_lib/Gas/Valves & Orifices/Orifice (G)  orifice_type=foundation.enum.constant_variable.variable  orifice_parameterization=fluids.gas.valves_orifices.enum.OrificeParameterization.Area  opening_characteristic=fluids.gas.valves_orifices.enum.OpeningCharacteristics.Linear  Cv_constant=4  Cv_max=4  L_Cv_TLU=0 : 0.2 : 1  Cv_TLU=[1e-06, .8, 1.6, 2.4, 3.2, 4]  xT_Cv=0.7  Kv_constant=3.6  Kv_max=3.6  L_Kv_TLU=0 : 0.2 : 1  Kv_TLU=[1e-06, .72, 1.44, 2.16, 2.88, 3.6]  xT_Kv=0.7  C_constant=12 l/(bar*s)  B_crit_constant=0.3  C_max=12 l/(bar*s)  B_crit_linear=0.3  L_C_TLU=0 : 0.2 : 1  C_TLU=[1e-05, 2.4, 4.8, 7.2, 9.6, 12] l/(bar*s)  B_crit_TLU=0.3 * ones(1, 6)  m=0.5  T_ref_C=293.15 K  rho_ref_C=1.185 kg/m^3  orifice_area_constant=1e-4 m^2  orifice_area_max=1963 mm^2  L_orifice_area_TLU=0 : 0.2 : 1  orifice_area_TLU=[1e-10, 2e-05, 4e-05, 6e-05, 8e-05, .0001] m^2  Cd=0.64  leakage_fraction=1e-6  smoothing_factor=0.01  B_lam=0.999  area=0.01 m^2
      settings: InternalSimscapePortConfiguration="{\"Bottom\":[],\"Left\":[{\"id\":\"A\",\"label\":\"A\",\"type\":\"foundation.gas.gas\"},{\"id\":\"L\",\"label\":\"L\",\"type\":\"input\"}],\"Right\":[{\"id\":\"B\",\"label\":\"B\",\"type\":\"foundation.gas.gas\"}],\"Top\":[]}"
  PS Gain : fl_lib/Physical Signals/Functions/PS Gain  Commented=on  gain=-100 Pa
  PS Terminator : fl_lib/Physical Signals/Sinks/PS Terminator
  PS Terminator1 : fl_lib/Physical Signals/Sinks/PS Terminator
  PS-Simulink Converter : nesl_utility/PS-Simulink Converter  PhysicalDomain=network_engine_domain  SubClassName=ps_output  LeftPortType=input  RightPortType=output  PseudoPeriodic=off  Frequencies=[]  VectorFormat=inherit  Unit=inherit  AffineConversion=off
  Pipe (G) : fl_lib/Gas/Elements/Pipe (G)  Commented=on  length=2 m  area=0.0001 m^2  Dh=0.1 m  length_add=1 m  roughness=15e-6 m  Re_lam=2000  Re_tur=4000  shape_factor=64  Nu_lam=3.66  p_I_specify=off  p_I_priority=High  p_I=0.101325 MPa  p_I_nominal_specify=off  p_I_nominal_unit=bar  p_I_nominal_value=1.5  T_I_specify=off  T_I_priority=High  T_I=293.15 K  T_I_nominal_specify=off  T_I_nominal_unit=K  T_I_nominal_value=1  rho_I_specify=off  rho_I_priority=None  rho_I=1.2 kg/m^3  rho_I_nominal_specify=off  rho_I_nominal_unit=kg/m^3  rho_I_nominal_value=1
  Pipe (G)2 : fl_lib/Gas/Elements/Pipe (G)  Commented=on  length=8.36 cm  area=3640 cm^2  Dh=1 cm  length_add=0.1 m  roughness=15e-6 m  Re_lam=2000  Re_tur=4000  shape_factor=64  Nu_lam=3.66  p_I_specify=on  p_I_priority=High  p_I=0.101325 MPa  p_I_nominal_specify=off  p_I_nominal_unit=MPa  p_I_nominal_value=1  T_I_specify=on  T_I_priority=High  T_I=293.15 K  T_I_nominal_specify=off  T_I_nominal_unit=K  T_I_nominal_value=1  rho_I_specify=off  rho_I_priority=None  rho_I=1.2 kg/m^3  rho_I_nominal_specify=off  rho_I_nominal_unit=kg/m^3  rho_I_nominal_value=1
  Reservoir (2P) : fl_lib/Two-Phase Fluid/Elements/Reservoir (2P)  pressure_spec=foundation.enum.ReservoirPressureSpec2P.Specified  reservoir_pressure=0.201325 MPa  reservoir_condensing_temperature=373.15 K  reservoir_evaporating_temperature=373.15 K  energy_spec=foundation.enum.ReservoirEnergySpec2P.Temperature  reservoir_temperature=280 K  reservoir_quality=0.5  reservoir_void_fraction=0.5  reservoir_enthalpy=1500 kJ/kg  reservoir_internal_energy=1500 kJ/kg  reservoir_subcooling=5 deltaK  reservoir_superheating=5 deltaK  area_A=0.01 m^2
  Reservoir (2P)1 : fl_lib/Two-Phase Fluid/Elements/Reservoir (2P)  pressure_spec=foundation.enum.ReservoirPressureSpec2P.Atmospheric  reservoir_pressure=0.51325 MPa  reservoir_condensing_temperature=373.15 K  reservoir_evaporating_temperature=373.15 K  energy_spec=foundation.enum.ReservoirEnergySpec2P.Temperature  reservoir_temperature=293.15 K  reservoir_quality=0.5  reservoir_void_fraction=0.5  reservoir_enthalpy=1500 kJ/kg  reservoir_internal_energy=1500 kJ/kg  reservoir_subcooling=5 deltaK  reservoir_superheating=5 deltaK  area_A=0.01 m^2
  Reservoir (TL) : fl_lib/Thermal Liquid/Elements/Reservoir (TL)  pressure_spec=foundation.enum.pressure_spec.specified  reservoir_pressure=0.201325 MPa  reservoir_temperature=293.15 K  area=0.01 m^2
  Reservoir (TL)1 : fl_lib/Thermal Liquid/Elements/Reservoir (TL)  pressure_spec=foundation.enum.pressure_spec.atmospheric  reservoir_pressure=0.101325 MPa  reservoir_temperature=293.15 K  area=0.01 m^2
  S1 : Subsystem
  S2 : Subsystem
  S3 : Subsystem
  S4 : Subsystem
      settings: PortSchema="{\"entries\":[{\"content\":{\"sides\":[{\"content\":{},\"type\":\"ConnectorPlacement.EquallySpacedRectSide\",\"uuid\":\"ecabe8b1-fc4e-4230-aeb9-96efa1b00fb1\"},{\"content\":{\"side\":\"RIGHT\"},\"type\":\"ConnectorPlacement.EquallySpacedRectSide\",\"uuid\":\"c3489f06-210d-4712-a62f-cf811e357432\"},{\"content\":{\"connectorIds\":[\"LConn1\"],\"side\":\"TOP\"},\"type\":\"ConnectorPlacement.EquallySpacedRectSide\",\"uuid\":\"e9362acc-cc64-4965-8c8e-b73e5511f057\"},{\"content\":{\"connectorIds\":[\"RConn1\"],\"side\":\"BOTTOM\"},\"type\":\"ConnectorPlacement.EquallySpacedRectSide\",\"uuid\":\"8047c48f-73de-4c30-9732-807ac22a5eff\"}]},\"type\":\"ConnectorPlacement.EquallySpacedConnector\",\"uuid\":\"942885bc-59c1-4140-9904-af1edff99dbd\"}],\"packageUris\":[\"http://schema.mathworks.com/mf0/Connector/R2020b\"],\"version\":\"1.0\"}"
  S5 : Subsystem
  S6 : Subsystem
  S7 : Subsystem
  S8 : Subsystem
  S9 : Subsystem
  Scope : Scope
  Simulink-PS Converter : nesl_utility/Simulink-PS Converter  Commented=on  PhysicalDomain=network_engine_domain  SubClassName=ps_input  LeftPortType=input  RightPortType=output  PseudoPeriodic=off  Frequencies=[]  NoiseDistribution=none  NoiseParameters=[]  Unit=1  AffineConversion=off  FilteringAndDerivatives=provide  SimscapeFilterOrder=1  InputFilterTimeConstant=0.001  UdotUserProvided=0
  Simulink-PS Converter1 : nesl_utility/Simulink-PS Converter  PhysicalDomain=network_engine_domain  SubClassName=ps_input  LeftPortType=input  RightPortType=output  PseudoPeriodic=off  Frequencies=[]  NoiseDistribution=none  NoiseParameters=[]  Unit=rpm  AffineConversion=off  FilteringAndDerivatives=provide  SimscapeFilterOrder=1  InputFilterTimeConstant=0.001  UdotUserProvided=0
  Simulink-PS Converter{2..3,5..10} (8 alike) : nesl_utility/Simulink-PS Converter  PhysicalDomain=network_engine_domain  SubClassName=ps_input  LeftPortType=input  RightPortType=output  PseudoPeriodic=off  Frequencies=[]  NoiseDistribution=none  NoiseParameters=[]  Unit=1  AffineConversion=off  FilteringAndDerivatives=provide  SimscapeFilterOrder=1  InputFilterTimeConstant=0.001  UdotUserProvided=0
  Simulink-PS Converter11 : nesl_utility/Simulink-PS Converter  PhysicalDomain=network_engine_domain  SubClassName=ps_input  LeftPortType=input  RightPortType=output  PseudoPeriodic=off  Frequencies=[]  NoiseDistribution=none  NoiseParameters=[]  Unit=K  AffineConversion=off  FilteringAndDerivatives=provide  SimscapeFilterOrder=1  InputFilterTimeConstant=0.001  UdotUserProvided=0
  Simulink-PS Converter12 : nesl_utility/Simulink-PS Converter  PhysicalDomain=network_engine_domain  SubClassName=ps_input  LeftPortType=input  RightPortType=output  PseudoPeriodic=off  Frequencies=[]  NoiseDistribution=none  NoiseParameters=[]  Unit=rpm  AffineConversion=off  FilteringAndDerivatives=provide  SimscapeFilterOrder=1  InputFilterTimeConstant=0.001  UdotUserProvided=0
  Simulink-PS Converter13 : nesl_utility/Simulink-PS Converter  PhysicalDomain=network_engine_domain  SubClassName=ps_input  LeftPortType=input  RightPortType=output  PseudoPeriodic=off  Frequencies=[]  NoiseDistribution=none  NoiseParameters=[]  Unit=Pa  AffineConversion=off  FilteringAndDerivatives=provide  SimscapeFilterOrder=1  InputFilterTimeConstant=0.001  UdotUserProvided=0
  Simulink-PS Converter4 : nesl_utility/Simulink-PS Converter  Commented=on  PhysicalDomain=network_engine_domain  SubClassName=ps_input  LeftPortType=input  RightPortType=output  PseudoPeriodic=off  Frequencies=[]  NoiseDistribution=none  NoiseParameters=[]  Unit=K  AffineConversion=off  FilteringAndDerivatives=filter  SimscapeFilterOrder=1  InputFilterTimeConstant=0.001  UdotUserProvided=0
  Solver Configuration1 : nesl_utility/Solver Configuration  PhysicalDomain=network_engine_domain  SubClassName=solver  LeftPortType=input  RightPortType=generic  Tones=[]  Harmonics=[]  SimulateNoise=off  Profile=off  UseLocalSampling=off  EnableSwitchedLinearOptims=on  FrequencyDomain=off  UseCCode=off  RelTol=0.001  AbsTol=0.001  MinStep=1e-09  ToWorkspace=off  RevertToSquareIcSolve=off  NumHomotopyIterations=100  PhasorMode=off  PhasorModeNumHarmonics=1  ConsistencySolver=NEWTON_XTOL_AFTER_FTOL  IndexReductionMethod=DerivativeReplacement  DoDC=off  ResidualTolerance=1e-09  ConsistencyTolSource=GLOBAL  ConsistencyAbsTol=0.001  ConsistencyRelTol=0.001  ConsistencyTolFactor=0.001  UseLocalSolver=off  LocalSolverChoice=NE_BACKWARD_EULER_ADVANCER  ResolveIndetEquations=on  FunctionEvalNumThread=1  LocalSolverSampleTime=0.001  DoFixedCost=off  MaxNonlinIter=3  MaxModeIter=2  ComputeImpulses=off  ImpulseIterations=2  LinearAlgebra=auto  LinearAlgebraNumThread=0  EquationFormulation=NE_TIME_EF  DelaysMemoryBudget=1024  AutomaticFiltering=on  FilteringTimeConstant=0.001  PartitionStorageMethod=AS_NEEDED  PartitionMemoryBudget=1024  PartitionMethod=ROBUST
  Thermal Liquid Properties (TL) : SimscapeFluids_lib/Thermal Liquid/Utilities/Thermal Liquid Properties (TL)  fluid_list=fluids.thermal_liquid.utilities.enum.thermal_liquid_fluid_list.water  concentration_param_EG=fluids.thermal_liquid.utilities.enum.thermal_liquid_concentration.volume_fraction  concentration_param_PG=fluids.thermal_liquid.utilities.enum.thermal_liquid_concentration.volume_fraction  c_mass_SW=3.5e-3  c_mass_EG=0.1  c_mass_PG=0.1  c_mass_GL=0.1  c_vol_EG=0.1  c_vol_PG=0.1  beta_const_EG=2.1791 GPa  beta_const_PG=2.1791 GPa  beta_const_GL=2.1791 GPa  p_min_EG=0.01 MPa  p_min_PG=0.01 MPa  p_min_GL=0.01 MPa  p_max_EG=50 MPa  p_max_PG=50 MPa  p_max_GL=50 MPa  p_atm=0.101325 MPa  properties_range_check=simscape.enum.assert.action.error
  Thermal Reference1 : fl_lib/Thermal/Thermal Elements/Thermal Reference  Commented=on
  Thermal Reference3 : fl_lib/Thermal/Thermal Elements/Thermal Reference  Commented=on
  Two-Phase Fluid Predefined Properties (2P) : SimscapeFluids_lib/Two-Phase Fluid/Utilities/Two-Phase Fluid Predefined Properties (2P)  fluid=fluids.two_phase_fluid.utilities.enum.Fluid.Water  p_atm=0.101325 MPa  properties_range_check=simscape.enum.assert.action.error  q_rev=0.01 Pa
  VSEC15_c200 (G)2 : SimscapeFluids_lib/Gas/Turbomachinery/Compressor (G)  parameterization=fluids.gas.turbomachinery.enum.CompressorParameterization.Tabulated  NDes=10000 rpm  piDes=7.5  mdotDes=33 kg/s  efficiencyType=fluids.gas.turbomachinery.enum.EfficiencyType.Analytical  efficiencyValue=0.8  etaMax=0.887  etaMin=0.5  mdotMaxEff=30 kg/s  piMaxEff=7  omega_TLU=VSEC15_c200_omega_TLU rpm  beta_TLU=0 : 1 / 5 : 1  pr_TLU=VSEC15_c200_pr_TLU  mdot_TLU=VSEC15_c200_mdot_TLU g/s  eta_TLU=VSEC15_c200_eta_TLU  SMFault=simscape.enum.assert.action.none  a=1.5  b=5  k=0.03  c=3  d=4  cCap=15  dCap=1  p_reference=0.101325 MPa  T_reference=288.15 K  mechanical_efficiency=0.98  area_A=0.002 m^2  area_B=0.002 m^2
      settings: InternalSimscapePortConfiguration="{\"Bottom\":[],\"Left\":[{\"id\":\"A\",\"label\":\"A\",\"type\":\"foundation.gas.gas\"},{\"id\":\"C\",\"label\":\"C\",\"type\":\"foundation.mechanical.rotational.rotational\"}],\"Right\":[{\"id\":\"B\",\"label\":\"B\",\"type\":\"foundation.gas.gas\"},{\"id\":\"R\",\"label\":\"R\",\"type\":\"foundation.mechanical.rotational.rotational\"},{\"id\":\"SM\",\"label\":\"SM\",\"type\":\"output\"}],\"Top\":[]}"
  VSEC15_c220 (G)1 : SimscapeFluids_lib/Gas/Turbomachinery/Compressor (G)  parameterization=fluids.gas.turbomachinery.enum.CompressorParameterization.Tabulated  NDes=10000 rpm  piDes=7.5  mdotDes=33 kg/s  efficiencyType=fluids.gas.turbomachinery.enum.EfficiencyType.Analytical  efficiencyValue=0.8  etaMax=0.887  etaMin=0.5  mdotMaxEff=30 kg/s  piMaxEff=7  omega_TLU=VSEC15_c220_omega_TLU rpm  beta_TLU=0 : 1 / 6 : 1  pr_TLU=VSEC15_c220_pr_TLU  mdot_TLU=VSEC15_c220_mdot_TLU g/s  eta_TLU=VSEC15_c220_eta_TLU  SMFault=simscape.enum.assert.action.none  a=1.5  b=5  k=0.03  c=3  d=4  cCap=15  dCap=1  p_reference=0.101325 MPa  T_reference=288.15 K  mechanical_efficiency=0.9  area_A=0.002 m^2  area_B=0.002 m^2
      settings: InternalSimscapePortConfiguration="{\"Bottom\":[],\"Left\":[{\"id\":\"A\",\"label\":\"A\",\"type\":\"foundation.gas.gas\"},{\"id\":\"C\",\"label\":\"C\",\"type\":\"foundation.mechanical.rotational.rotational\"}],\"Right\":[{\"id\":\"B\",\"label\":\"B\",\"type\":\"foundation.gas.gas\"},{\"id\":\"R\",\"label\":\"R\",\"type\":\"foundation.mechanical.rotational.rotational\"},{\"id\":\"SM\",\"label\":\"SM\",\"type\":\"output\"}],\"Top\":[]}"
  Connection Port : PMIOPort  Side=Left
  Output : Outport
  Output1 : Outport  Port=2
  wires:
  Constant11/1 -> Inlet/Outlet1/1(T_amb_K), Simulink-PS Converter11/1
  20231018_14_31_59_ATP/1(current) -> 1-stake cooling will replace this lookup table/1, 1-D Lookup Table/1
  Constant10/1 -> Simulink-PS Converter13/1, Inlet/Outlet1/2(p_amb_Pa)
  1-D Lookup Table/1 -> Simulink-PS Converter/1
  1-stake cooling will replace this lookup table/1 -> Simulink-PS Converter4/1
  Constant/1 -> Simulink-PS Converter2/1
  Constant2/1 -> Simulink-PS Converter3/1
  In1/1 -> Bus Selector/1
  Bus Selector/4 -> Gain1/1  "<EAT_LP_bypass_Valve>"
  Bus Selector/1 -> Simulink-PS Converter1/1  "<EAC_LP_RPM>"
  Bus Selector/2 -> Gain/1  "<LP_Bleed_valve>"
  Gain/1 -> Simulink-PS Converter5/1
  Bus Selector/3 -> Simulink-PS Converter6/1  "<EAT_LP_VNT>"
  In2/1 -> Bus Selector1/1
  Bus Selector1/1 -> Gain3/1  "<HP_Bleed_valve1>"
  Bus Selector1/4 -> Gain2/1  "<EAT_HP_bypass_Valve1>"
  Bus Selector1/2 -> Simulink-PS Converter10/1  "<EAT_HP_VNT1>"
  Gain1/1 -> Simulink-PS Converter7/1
  Gain2/1 -> Simulink-PS Converter8/1
  Bus Selector1/3 -> Simulink-PS Converter12/1  "<EAC_HP_RPM1>"
  Gain3/1 -> Simulink-PS Converter9/1
  [EAC001] -> Bus Selector2/1
  [EAC201] -> Bus Selector3/1
  [TB701] -> Bus Selector4/1
  [TB721] -> Bus Selector5/1
  Bus Selector2/1 -> Bus Creator/1  "<PT-C-001>"
  Bus Selector2/2 -> Bus Creator/2  "<TT-C-001>"
  Bus Selector2/3 -> Bus Creator/3  "<FT-C001>"
  Bus Selector3/1 -> Bus Creator/4  "<PT-C-201>"
  Bus Selector4/1 -> Bus Creator/5  "<PT701>"
  Bus Selector5/1 -> Bus Creator/6  "<PT721>"
  Bus Creator/1 -> Output/1
  [EAC201] -> Bus Selector6/1
  [EAC211] -> Bus Selector7/1
  [TB511] -> Bus Selector8/1
  [stake411] -> Bus Selector9/1
  Bus Selector6/1 -> Bus Creator1/1  "<PT-C-201>"
  Bus Selector6/3 -> Bus Creator1/3  "<TT-C-201>"
  Bus Selector7/1 -> Bus Creator1/4  "<PT-C-211>"
  Bus Selector8/1 -> Bus Creator1/5  "<PT511>"
  Bus Selector6/2 -> Bus Creator1/2  "<FT-C-201>"
  Bus Selector9/1 -> Bus Creator1/6  "<PT-C-411>"
  Bus Creator1/1 -> Output1/1
  PS-Simulink Converter/1 -> Scope/1
  connections:
  Simulink-PS Converter12/RConn1 -- Ideal Angular Velocity Source2/RConn1
  Simulink-PS Converter/RConn1 -- PS Gain/LConn1
  H.P Turbine1/RConn1 -- Orifice (G)6/RConn1 -- S5/LConn1 -- Orifice (G)3/RConn1
  Mechanical Rotational Reference2/LConn1 -- LPTurbine (G)2/RConn2
  Simulink-PS Converter6/RConn1 -- LPTurbine (G)2/LConn3
  S2/RConn1 -- Orifice (G)6/LConn1 -- VSEC15_c220 (G)1/LConn1
  Mechanical Rotational Reference6/LConn1 -- VSEC15_c200 (G)2/LConn2
  Controlled Reservoir (G)/LConn1 -- S7/RConn1
  VSEC15_c220 (G)1/RConn2 -- H.P Turbine1/LConn2 -- Ideal Angular Velocity Source2/LConn1
  Thermal Reference1/LConn1 -- Controlled Temperature Source/RConn2
  PS Gain/RConn1 -- Controlled Pressure Source (G)1/LConn2
  Inlet/Outlet1/RConn1 -- S1/LConn1
  Mechanical Rotational Reference1/LConn1 -- H.P Turbine1/RConn2
  Mechanical Rotational Reference5/LConn1 -- VSEC15_c220 (G)1/LConn2
  Controlled Temperature Source/LConn1 -- INTER6511/RConn1
  VSEC15_c200 (G)2/RConn3 -- PS Terminator/LConn1
  HC2/RConn1 -- INTER6511/RConn3
  Controlled Temperature Source/RConn1 -- Inlet/Outlet1/RConn3
  C2/RConn1 -- INTER6511/RConn2
  VSEC15_c220 (G)1/RConn1 -- S6/LConn1
  S1/RConn1 -- VSEC15_c200 (G)2/LConn1
  VSEC15_c200 (G)2/RConn1 -- S2/LConn1
  VSEC15_c220 (G)1/RConn3 -- PS Terminator1/LConn1
  S8/RConn1 -- Orifice (G)3/LConn1 -- H.P Turbine1/LConn1
  Simulink-PS Converter10/RConn1 -- H.P Turbine1/LConn3
  Controlled Temperature Source1/LConn1 -- Pipe (G)2/LConn2
  Thermal Reference3/LConn1 -- Controlled Temperature Source1/RConn2
  Simulink-PS Converter4/RConn1 -- Controlled Temperature Source1/RConn1
  S4/LConn1 -- Orifice (G)2/LConn1
  Orifice (G)1/LConn1 -- Orifice (G)5/LConn1 -- S3/RConn1
  VSEC15_c200 (G)2/RConn2 -- Ideal Angular Velocity Source1/LConn1 -- LPTurbine (G)2/LConn2
  Mechanical Rotational Reference3/LConn1 -- Ideal Angular Velocity Source2/RConn2
  Mechanical Rotational Reference4/LConn1 -- Ideal Angular Velocity Source1/RConn2
  Simulink-PS Converter1/RConn1 -- Ideal Angular Velocity Source1/RConn1
  Simulink-PS Converter2/RConn1 -- Orifice (G)2/LConn2
  Simulink-PS Converter3/RConn1 -- Orifice (G)1/LConn2
  Simulink-PS Converter5/RConn1 -- Orifice (G)4/LConn2
  Simulink-PS Converter7/RConn1 -- Orifice (G)6/LConn2
  Simulink-PS Converter8/RConn1 -- Orifice (G)5/LConn2
  Simulink-PS Converter9/RConn1 -- Orifice (G)3/LConn2
  S7/LConn1 -- Orifice (G)4/RConn1 -- LPTurbine (G)2/RConn1
  Orifice (G)4/LConn1 -- S5/RConn1 -- LPTurbine (G)2/LConn1
  Orifice (G)2/RConn1 -- S8/LConn1 -- Solver Configuration1/RConn1 -- Orifice (G)5/RConn1
  Orifice (G)1/RConn1 -- S9/LConn1
  Simulink-PS Converter11/RConn1 -- Controlled Reservoir (G)/RConn1
  Simulink-PS Converter13/RConn1 -- Controlled Reservoir (G)/RConn2
  S3/LConn1 -- Heat Exchanger (G-TL)/LConn2
  S6/RConn1 -- Heat Exchanger (G-TL)/LConn1
  S4/RConn1 -- Flow Resistance (G)/RConn1
  Flow Resistance (G)/LConn1 -- S9/RConn1
  Reservoir (TL)/LConn1 -- Thermal Liquid Properties (TL)/RConn1 -- Condenser Evaporator (TL-2P)/LConn1
  Condenser Evaporator (TL-2P)/LConn2 -- Heat Exchanger (G-TL)/RConn1
  Reservoir (2P)/LConn1 -- Condenser Evaporator (TL-2P)/RConn1
  Reservoir (2P)1/LConn1 -- Two-Phase Fluid Predefined Properties (2P)/RConn1 -- Condenser Evaporator (TL-2P)/RConn2
  Heat Exchanger (G-TL)/RConn2 -- Reservoir (TL)1/LConn1
  Condenser Evaporator (TL-2P)/LConn3 -- PS-Simulink Converter/LConn1

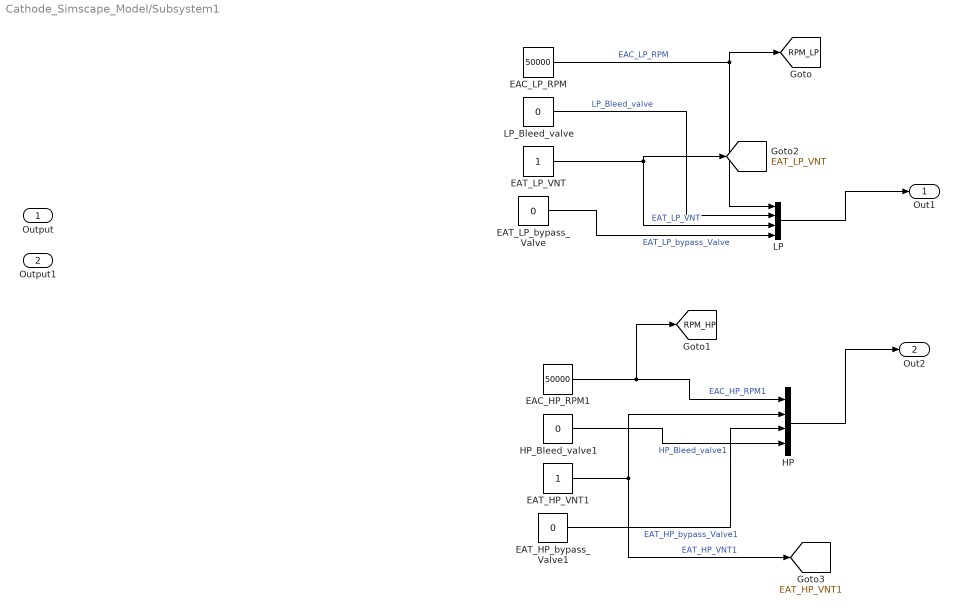
== system Cathode_Simscape_Model/Subsystem1 ==
  Output : Inport
  Output1 : Inport  Port=2
  EAC_HP_RPM1 : Constant  Value=50000
  EAC_LP_RPM : Constant  Value=50000
  EAT_HP_VNT1 : Constant
  EAT_HP_bypass_Valve1 : Constant  Value=0
  EAT_LP_VNT : Constant
  EAT_LP_bypass_Valve : Constant  Value=0
  HP : BusCreator  Inputs=4
  HP_Bleed_valve1 : Constant  Value=0
  LP : BusCreator  Inputs=4
  LP_Bleed_valve : Constant  Value=0
  Out1 : Outport
  Out2 : Outport  Port=2
  tag scope: EAT_HP_VNT1=global, EAT_LP_VNT=global, RPM_HP=global, RPM_LP=global
  wires:
  EAT_HP_bypass_Valve1/1 -> HP/3  "EAT_HP_bypass_Valve1"
  EAT_LP_bypass_Valve/1 -> LP/4  "EAT_LP_bypass_Valve"
  EAC_HP_RPM1/1 -> [RPM_HP], HP/1  "EAC_HP_RPM1"
  EAT_LP_VNT/1 -> LP/3, [EAT_LP_VNT]  "EAT_LP_VNT"
  EAC_LP_RPM/1 -> LP/1, [RPM_LP]  "EAC_LP_RPM"
  HP_Bleed_valve1/1 -> HP/4  "HP_Bleed_valve1"
  LP_Bleed_valve/1 -> LP/2  "LP_Bleed_valve"
  EAT_HP_VNT1/1 -> [EAT_HP_VNT1], HP/2  "EAT_HP_VNT1"
  LP/1 -> Out1/1
  HP/1 -> Out2/1

== system Cathode_Simscape_Model/Subsystem/20231018_14_31_59_ATP ==
  Demux : Demux  Tag=STV Demux  Outputs=1
      settings: DisplayOption=none
  FromWs : FromWorkspace  Tag=STV FromWs  VariableName=tuvar
      SigBuilderData=|
      | common.afterFinalStr = 'Extrapolate'
      | common.sampleTime = 0
      | dataSet.timeRange = [0 4735]
      | dataSet.name = 'Sheet1'
      | sbobj.Groups.Name = 'Sheet1'
      | sbobj.Groups.Signals.Name = 'current'
      | sbobj.Groups.Signals.XData = [0 125 125 270 270 375 375 1000 1000 1020 1080 1100 1200 1230 1260 1270 1320 1340 1390 1405 1455 1475 1525 1565 3990 4000 4030 4090 4130 4245 4270 4345 4355 4385 4395 4735]
      | sbobj.Groups.Signals.YData = [100 101 151 151 201 200 350 350 100 200 200 300 300 45 45 50 50 200 200 300 300 100 100 420 420 340 420 260 340 340 50 50 45 45 5 5]
      | sbobj.Groups.TimeRange = [0 4735]
  current : Outport  Tag=STV Outport
  wires:
  Demux/1 -> current/1
  FromWs/1 -> Demux/1
